simulink model "MR_CIGRE_RESISTIVO"  (R2017b)
settings: Solver=ode23tb  StartTime=0.0  StopTime=t_sim  RelTol=1e-4
values from neighbouring files (symbols this model uses):
  Cdc_Bat1 = 2E-3    (= 0.002)    [Dados_de_Bat_1.m]
  Cf_Bat1 = 5E-6    (= 5e-06)    [Dados_de_Bat_1.m]
  I_max_Bat1 = 1.5*Is_bat1*sqrt(2)    [Dados_de_Bat_1.m]
  Is_bat1 = Sb_Bat1 / (sqrt(3)*Vs2)    [Dados_de_Bat_1.m]
  K_iff_Bat1 = 0    [Dados_de_Bat_1.m]
  Kcij = Rfsj*(2*sig*w_ij*(Tpj + Tfsj)-1)    (= 3.9715)    [Dados_de_Bat_1.m]
  Ki_Bat1 = (R_Bat1+ron_Bat1)/ti_Bat1    (= 201.76)    [Dados_de_Bat_1.m]
  Kp_Bat1 = L_Bat1/ti_Bat1    (= 2.7)    [Dados_de_Bat_1.m]
  Kv_Bat1 = 0.75    [Dados_de_Bat_1.m]
  Kvi_DC = 25*Kvp_DC    (= 7.5)    [Dados_de_Bat_1.m]
  Kvp_DC = 0.3    [Dados_de_Bat_1.m]
  L_10_18 = imag(ug3)*C_10_18    [Dados_de_Linhas.m]
  L_12_13 = imag(ug3)*C_12_13    [Dados_de_Linhas.m]
  L_13_14 = imag(ug3)*C_13_14    [Dados_de_Linhas.m]
  L_14_15 = imag(ug3)*C_14_15    [Dados_de_Linhas.m]
  L_1_2 = imag(ug1)*C_1_2    [Dados_de_Linhas.m]
  L_2_3 = imag(ug1)*C_2_3    [Dados_de_Linhas.m]
  L_3_11 = imag(ug3)*C_3_11    [Dados_de_Linhas.m]
  L_3_4 = imag(ug1)*C_3_4    [Dados_de_Linhas.m]
  L_4_12 = imag(ug3)*C_4_12    [Dados_de_Linhas.m]
  L_4_5 = imag(ug1)*C_4_5    [Dados_de_Linhas.m]
  L_5_6 = imag(ug1)*C_5_6    [Dados_de_Linhas.m]
  L_6_16 = imag(ug3)*C_6_16    [Dados_de_Linhas.m]
  L_6_7 = imag(ug1)*C_6_7    [Dados_de_Linhas.m]
  L_7_8 = imag(ug1)*C_7_8    [Dados_de_Linhas.m]
  L_8_9 = imag(ug1)*C_8_9    [Dados_de_Linhas.m]
  L_9_10 = imag(ug1)*C_9_10    [Dados_de_Linhas.m]
  L_9_17 = imag(ug3)*C_9_17    [Dados_de_Linhas.m]
  L_Bat1 = 1.35E-3    (= 0.00135)    [Dados_de_Bat_1.m]
  L_Bat2 = 1.35E-3    (= 0.00135)    [Dados_de_Bat_2.m]
  L_Virt_Bat1 = 3e-3    (= 0.003)    [Dados_de_Bat_1.m]
  L_Virt_Bat2 = 3.0E-3    (= 0.003)    [Dados_de_Bat_2.m]
  LC_Bat2 = 1e-16    [Dados_de_Bat_2.m]
  Lfsj = 4e-3    (= 0.004)    [Dados_de_Bat_1.m]
  LPF_Ci_Bat1 = 8000    [Dados_de_Bat_1.m]
  LPF_Ci_Bat2 = 5000    [Dados_de_Bat_2.m]
  LPF_Cv_Bat1 = 3000    [Dados_de_Bat_1.m]
  LPF_Q_Bat1 = 3*2*pi()    [Dados_de_Bat_1.m]
  m_Bat1 = 0.05    [Dados_de_Bat_1.m]
  n_Bat1 = 0.05    [Dados_de_Bat_1.m]
  PQ_ref_taxavar_bat1 = 0.5    [Dados_de_Bat_1.m]
  R_10_18 = real(ug3)*C_10_18    [Dados_de_Linhas.m]
  R_12_13 = real(ug3)*C_12_13    [Dados_de_Linhas.m]
  R_13_14 = real(ug3)*C_13_14    [Dados_de_Linhas.m]
  R_14_15 = real(ug3)*C_14_15    [Dados_de_Linhas.m]
  R_1_2 = real(ug1)*C_1_2    [Dados_de_Linhas.m]
  R_2_3 = real(ug1)*C_2_3    [Dados_de_Linhas.m]
  R_3_11 = real(ug3)*C_3_11    [Dados_de_Linhas.m]
  R_3_4 = real(ug1)*C_3_4    [Dados_de_Linhas.m]
  R_4_12 = real(ug3)*C_4_12    [Dados_de_Linhas.m]
  R_4_5 = real(ug1)*C_4_5    [Dados_de_Linhas.m]
  R_5_6 = real(ug1)*C_5_6    [Dados_de_Linhas.m]
  R_6_16 = real(ug3)*C_6_16    [Dados_de_Linhas.m]
  R_6_7 = real(ug1)*C_6_7    [Dados_de_Linhas.m]
  R_7_8 = real(ug1)*C_7_8    [Dados_de_Linhas.m]
  R_8_9 = real(ug1)*C_8_9    [Dados_de_Linhas.m]
  R_9_10 = real(ug1)*C_9_10    [Dados_de_Linhas.m]
  R_9_17 = real(ug3)*C_9_17    [Dados_de_Linhas.m]
  R_Bat1 = 0.1    [Dados_de_Bat_1.m]
  R_Virt_Bat1 = 0    [Dados_de_Bat_1.m]
  R_Virt_Bat2 = 0    [Dados_de_Bat_2.m]
  Rb_bat1 = (N_cell_serie * Rb_cell) / N_string_cell    (= 0.153333333333)    [Dados_de_Bat_1.m]
  RC_Bat2 = 1e-16    [Dados_de_Bat_2.m]
  Rfsj = 0.03    [Dados_de_Bat_1.m]
  ron_Bat1 = 0.88E-3    (= 0.00088)    [Dados_de_Bat_1.m]
  Vdc_Bat1 = 800    [Dados_de_Bat_1.m]
  Voc_bat1 = N_cell_serie * Voc_cell    (= 180)    [Dados_de_Bat_1.m]
  z_Bat1 = z_gk    [Dados_de_Bat_1.m]
undefined symbols (not defined in the file or in its folder): BAT1_CONT, BAT2_CONT, Cdc, Cf, cont_fre, cont_ten, f0, Imax_solar1, Imax_solar2, Ki_interm, Kie, Kiw, Kp_cp, Kp_cr, Kp_interm, Kpe, Kpw, L, LPF_P_Bat1, LPF_P_Interm, LPF_Vdc, P_Solar1, P_Solar2, PQ_ref_time_bat1, Pref_Bat1, Qref_Bat1, Qref_Solar, R, ron, Sb_Bat1, Sb_ger, Sb_sol1, Sb_sol2, t_atraso, t_CS_ini, TDR1, TDR11, TDR15, TDR16, TDR17, TDR18, ti_cp, ti_cr, tilha, TLR11, TLR15, TLR16, TLR17, TLR18, tsinc, Vdc, vref1, Vref_sec, Vs1, Vs2, w0, wref_sec
libraries: powerlib x158, powerlib_meascontrol x59, re_lib x2, simulink x1
(part 4 of 4)

== system MR_CIGRE_RESISTIVO/Banco de Baterias_2/Referencia de  Corrente ==
  Id_feed : Inport
  Iq_feed : Inport  Port=2
  Sw_Mode : Inport  Port=3
  Id_supp : Inport  Port=4
  Iq_supp : Inport  Port=5
  LPF2 : TransferFcn  Denominator=[1/(LPF_Cv_Bat1) 1]
  LPF4 : TransferFcn  Denominator=[1/(LPF_Cv_Bat1) 1]
  Switch : Switch  Criteria=u2 > Threshold
  Switch1 : Switch  Criteria=u2 > Threshold
  Id_ref : Outport
  Iq_ref : Outport  Port=2
  wires:
  Sw_Mode/1 -> Switch/2, Switch1/2
  Switch/1 -> LPF4/1
  Switch1/1 -> LPF2/1
  Id_feed/1 -> Switch/1
  Id_supp/1 -> Switch/3
  Iq_feed/1 -> Switch1/1
  Iq_supp/1 -> Switch1/3
  LPF2/1 -> Iq_ref/1
  LPF4/1 -> Id_ref/1

== system MR_CIGRE_RESISTIVO/Banco de Baterias_2/Referência de Potencia ==
  note: Mudança de referência: no sincronismo (sinc=1)
  note: Ref. Potencia em rampa p.u.
  sinc : Inport
  Pref_bat : Inport  Port=2
  Qref_bat : Inport  Port=3
  Pgd : Inport  Port=4
  Qgd : Inport  Port=5
  Data Store Memory : DataStoreMemory  DataStoreName=Qr  ReadBeforeWriteMsg=warning  WriteAfterWriteMsg=warning  WriteAfterReadMsg=warning  ShowAdditionalParam=off  OutDataTypeStr=double
  Data Store Memory1 : DataStoreMemory  DataStoreName=Pr  ReadBeforeWriteMsg=warning  WriteAfterWriteMsg=warning  WriteAfterReadMsg=warning  VectorParams1D=off  ShowAdditionalParam=off  OutDataTypeStr=double
  Product1 : Product
  Product2 : Product
  Rate Limiter : RateLimiter  RisingSlewLimit=PQ_ref_taxavar_bat1*Sb_Bat1  FallingSlewLimit=-PQ_ref_taxavar_bat1*Sb_Bat1  SampleTimeMode=inherited
  Rate Limiter1 : RateLimiter  RisingSlewLimit=PQ_ref_taxavar_bat1*Sb_Bat1  FallingSlewLimit=-PQ_ref_taxavar_bat1*Sb_Bat1  SampleTimeMode=inherited
  Referência Fonte : MATLAB Function  TreatAsAtomicUnit=on
  Time_init_ref : Step  Time=PQ_ref_time_bat1  SampleTime=0
  Prefbat : Outport
  Qrefbat : Outport  Port=2
  wires:
  Referência Fonte/1(Prefbat) -> Prefbat/1
  Referência Fonte/2(Qrefbat) -> Qrefbat/1
  sinc/1 -> Referência Fonte/5(sinc)
  Pgd/1 -> Referência Fonte/3(p)
  Qgd/1 -> Referência Fonte/4(q)
  Product2/1 -> Rate Limiter1/1
  Time_init_ref/1 -> Product1/2, Product2/1
  Qref_bat/1 -> Product2/2
  Product1/1 -> Rate Limiter/1
  Pref_bat/1 -> Product1/1
  Rate Limiter/1 -> Referência Fonte/1(Pref_bat)
  Rate Limiter1/1 -> Referência Fonte/2(Qref_bat)

== system MR_CIGRE_RESISTIVO/PCC/Ilhamento// Sincronização ==
  sinc : Inport
  Display : Display
  Display1 : Display
  Display3 : Display
  Ilhamento Chave fechada para chave aberta em tilha : Step  Time=tilha  Before=1  After=0  SampleTime=0
  Switch : Switch  Criteria=u2 > Threshold
  sinc=1 : Constant
  "Ch " : Outport
  wires:
  Ilhamento Chave fechada para chave aberta em tilha/1 -> Switch/3, Display3/1
  sinc=1/1 -> Switch/1, Display/1
  Switch/1 -> "Ch "/1, Display1/1
  sinc/1 -> Switch/2

== system MR_CIGRE_RESISTIVO/Sincronização/Microrrede ==
  Vabc : Inport
  Gain4 : Gain  Gain=1/(Vs2*sqrt(2))
  PLL (3ph) : powerlib_meascontrol/PLL/PLL (3ph)  Fmin=45  Par_Init="[0  60]"  ParK=[180, 3200, 1]  TcD=5E-5  MaxRateChangeFreq=12  FilterCutOffFreq=25  Ts=5E-5  AGC=on
  Sequence Analyzer : powerlib_meascontrol/Measurements/Sequence Analyzer  Freq=60  n=1  seq=Positive  InInit=[1, 0]  Ts=0
      settings: SourceProductName=Simscape Power Systems  SourceProductBaseCode=PS
  Ang : Outport
  |V| : Outport  Port=2
  f : Outport  Port=3
  wires:
  Vabc/1 -> Sequence Analyzer/1, PLL (3ph)/1
  PLL (3ph)/1 -> f/1
  Sequence Analyzer/2 -> Ang/1
  Gain4/1 -> |V|/1
  Sequence Analyzer/1 -> Gain4/1

== system MR_CIGRE_RESISTIVO/Sincronização/Rede Principal ==
  Vabc : Inport
  Gain4 : Gain  Gain=1/(Vs2*sqrt(2))
  PLL (3ph) : powerlib_meascontrol/PLL/PLL (3ph)  Fmin=45  Par_Init="[0  60]"  ParK=[180, 3200, 1]  TcD=5E-5  MaxRateChangeFreq=12  FilterCutOffFreq=25  Ts=5E-5  AGC=on
  Sequence Analyzer : powerlib_meascontrol/Measurements/Sequence Analyzer  Freq=60  n=1  seq=Positive  InInit=[1, 0]  Ts=0
      settings: SourceProductName=Simscape Power Systems  SourceProductBaseCode=PS
  f : Outport
  |V| : Outport  Port=2
  Ang : Outport  Port=3
  wires:
  Vabc/1 -> Sequence Analyzer/1, PLL (3ph)/1
  PLL (3ph)/1 -> f/1
  Sequence Analyzer/2 -> Ang/1
  Gain4/1 -> |V|/1
  Sequence Analyzer/1 -> Gain4/1

== system MR_CIGRE_RESISTIVO/Solar_1/Controle Corrente ==
  Idref : Inport
  Iqref : Inport  Port=2
  Vsd : Inport  Port=3
  Vsq : Inport  Port=4
  Id : Inport  Port=5
  Iq : Inport  Port=6
  w : Inport  Port=7
  Vdc/2 : Inport  Port=8
  Controle d : TransferFcn  Numerator=[Kp_interm Ki_interm]  Denominator=[1 0]
  Controle q : TransferFcn  Numerator=[Kp_interm Ki_interm]  Denominator=[1 0]
  Divide : Product  Inputs=*/
  Divide1 : Product  Inputs=/*
  L*w0*Id : Gain  Gain=L_Bat2
  L*w0*Iq : Gain  Gain=L_Bat2
  LPF1 : TransferFcn  Commented=through  Denominator=[1/(LPF_Ci_Bat2) 1]
  LPF2 : TransferFcn  Commented=through  Denominator=[1/(LPF_Ci_Bat2) 1]
  Saturation : Saturate  UpperLimit=1  LowerLimit=-1
  Saturation1 : Saturate  UpperLimit=1  LowerLimit=-1
  Sum1 : Sum  Inputs=-+|
  Sum2 : Sum  Inputs=+|+|-
  Sum3 : Sum  Inputs=|+-
  Sum4 : Sum  Inputs=+|+|+
  d : Product  Inputs=**
  q : Product  Inputs=**
  Md : Outport
  Mq : Outport  Port=2
  wires:
  Vsd/1 -> Sum2/1
  Saturation1/1 -> Md/1
  Saturation/1 -> Mq/1
  Sum2/1 -> Divide/1
  Iq/1 -> d/2, Sum3/2
  Iqref/1 -> Sum3/1
  w/1 -> d/1, q/2
  q/1 -> L*w0*Id/1
  Sum1/1 -> Controle d/1
  L*w0*Iq/1 -> Sum2/3
  Vdc/2/1 -> Divide1/1, Divide/2
  d/1 -> L*w0*Iq/1
  Idref/1 -> Sum1/2
  Sum4/1 -> Divide1/2
  Sum3/1 -> Controle q/1
  Controle d/1 -> Sum2/2
  Controle q/1 -> Sum4/2
  L*w0*Id/1 -> Sum4/1
  Id/1 -> q/1, Sum1/1
  Vsq/1 -> Sum4/3
  Divide1/1 -> LPF1/1
  Divide/1 -> LPF2/1
  LPF2/1 -> Saturation1/1
  LPF1/1 -> Saturation/1

== system MR_CIGRE_RESISTIVO/Solar_1/Controle Potencia  ==
  note: Anti Windup
  note: Anti Windup
  Q_ref : Inport
  Q : Inport  Port=2
  Vdc : Inport  Port=3
  Gain : Gain  Gain=Kp_cp
  Gain1 : Gain  Gain=Kp_cr
  Gain2 : Gain  Gain=Kp_cr
  Gain3 : Gain  Gain=1/Kp_cp
  Gain4 : Gain  Gain=Kp_cp
  Gain5 : Gain  Gain=-1
  Gain6 : Gain  Gain=1/Kp_cp
  Gain7 : Gain  Gain=-1
  Integrador d : TransferFcn  Denominator=[ti_cp 0]
  Integrador d1 : TransferFcn  Denominator=[ti_cr 0]
  Pref1 : Constant  Value=Vdc
  Referencia de  Corrente : Subsystem
  Sum1 : Sum  Inputs=+-|
  Sum10 : Sum  Inputs=+-
  Sum2 : Sum  Inputs=+-|
  Sum3 : Sum  Inputs=||+|+
  Sum4 : Sum  Inputs=+|+||
  Sum5 : Sum  Inputs=+|-
  Sum6 : Sum  Inputs=-+
  Sum8 : Sum  Inputs=+|-
  Id_ref : Outport
  Iq_ref : Outport  Port=2
  wires:
  Vdc/1 -> Sum1/2
  Pref1/1 -> Sum1/1
  Integrador d1/1 -> Sum3/2
  Sum2/1 -> Gain5/1
  Q_ref/1 -> Sum2/1
  Q/1 -> Sum2/2
  Gain3/1 -> Sum6/1
  Referencia de  Corrente/1(Id_lim) -> Id_ref/1, Sum5/2
  Sum4/1 -> Sum5/1, Referencia de  Corrente/1(Id_ref)
  Gain6/1 -> Sum10/2
  Sum8/1 -> Gain6/1
  Sum5/1 -> Gain3/1
  Referencia de  Corrente/2(Iq_lim) -> Iq_ref/1, Sum8/2
  Sum3/1 -> Referencia de  Corrente/2(Iq_ref), Sum8/1
  Gain1/1 -> Integrador d1/1
  Sum10/1 -> Gain1/1
  Gain2/1 -> Sum3/1
  Gain/1 -> Integrador d/1
  Sum6/1 -> Gain/1
  Sum1/1 -> Gain7/1
  Gain4/1 -> Sum4/2
  Gain5/1 -> Gain2/1, Sum10/1
  Gain7/1 -> Gain4/1, Sum6/2
  Integrador d/1 -> Sum4/1

== system MR_CIGRE_RESISTIVO/Solar_1/Elo CC ==
  CM1 : powerlib/Measurements/Current Measurement  PhasorSimulation=off  OutputType=Complex  PSBequivalent=0
  P : Product  Inputs=**
  Parallel RLC Branch : powerlib/Elements/Parallel RLC Branch  LConnTagsString=a  RConnTagsString=__new0  BranchType=C  Resistance=10000000  Inductance=0  SetiL0=off  InitialCurrent=0  Capacitance=Cdc  Setx0=on  InitialVoltage=710  Measurements=None
  Unit Delay1 : UnitDelay  Commented=through  InitialCondition=700  SampleTime=1E-6
  VM1 : powerlib/Measurements/Voltage Measurement  PhasorSimulation=off  OutputType=Complex  PSBequivalent=0
  + in : PMIOPort  Port=1  Side=Left
  - in : PMIOPort  Port=2  Side=Left
  + out : PMIOPort  Port=3  Side=Right
  - out : PMIOPort  Port=4  Side=Right
  Vdc : Outport
  Pout : Outport  Port=2
  wires:
  VM1/1 -> P/2, Unit Delay1/1
  P/1 -> Pout/1
  CM1/1 -> P/1
  Unit Delay1/1 -> Vdc/1
  connections:
  VM1/LConn2 -- - out/RConn1 -- Parallel RLC Branch/RConn1 -- - in/RConn1
  VM1/LConn1 -- CM1/LConn1 -- + in/RConn1 -- Parallel RLC Branch/LConn1
  + out/RConn1 -- CM1/RConn1

== system MR_CIGRE_RESISTIVO/Solar_1/Fonte Fotovoltaica ==
  CM1 : powerlib/Measurements/Current Measurement  PhasorSimulation=off  OutputType=Complex  PSBequivalent=0
  P : Product  Inputs=**
  PV Array : re_lib/Solar/PV Array  Npar=P_Solar1/3000  Nser=10  PlotType=array @ 1000 W/m2 & specified temperatures  S_vec="[ 1000  500  100 ]"  Temp_C_vec="[ 45 25  ]"  ModuleName=Canadian Solar CS6X-300P  PlotWhenSelected=off  Pm=299.63  Ncell=72  Voc=44.6  Isc=8.87  Vm=36.1  Im=8.3  beta_Voc_pc=-0.395  alpha_Isc_pc=0.052999  beta_Voc=-0.17617  alpha_Isc=0.004701  IL=8.9088  I0=9.446e-10  nI=1.0506  Rsh=262.4171  Rs=0.34354  BAL=off  Tc=1e-6  Tfilter=5e-5
  Pref3 : Constant  Value=1000
  Pref4 : Constant  Value=25
  Pref5 : Constant  Value=0.5157
  Two-Quadrant DC/DC Converter : powerlib/Power Electronics/Two-Quadrant DC//DC Converter  ModelType=Average model (D-controlled)  Ron=1e-3  Rs=1e6  Cs=inf  Vforward=[0,0]  Ron_Diode=1e-3  Rs_Diode=1e6  Cs_Diode=inf  Vf_Diode=1e-3  Rs_CurrentSource=inf
      settings: SourceProductName=Simscape Power Systems  SourceProductBaseCode=PS
  VM1 : powerlib/Measurements/Voltage Measurement  PhasorSimulation=off  OutputType=Complex  PSBequivalent=0
  VM3 : powerlib/Measurements/Voltage Measurement  PhasorSimulation=off  OutputType=Complex  PSBequivalent=0
  w3 : Scope
  + out : PMIOPort  Port=1  Side=Left
  - out : PMIOPort  Port=2  Side=Left
  V_fv : Outport
  P_fv : Outport  Port=2
  wires:
  Pref3/1 -> PV Array/1
  Pref5/1 -> Two-Quadrant DC/DC Converter/1
  VM3/1 -> w3/1
  Pref4/1 -> PV Array/2
  VM1/1 -> V_fv/1, P/2
  CM1/1 -> P/1
  P/1 -> P_fv/1
  connections:
  PV Array/RConn2 -- VM3/LConn2 -- VM1/LConn2 -- - out/RConn1 -- Two-Quadrant DC/DC Converter/RConn2
  VM3/LConn1 -- PV Array/RConn1 -- Two-Quadrant DC/DC Converter/LConn1
  CM1/LConn1 -- Two-Quadrant DC/DC Converter/RConn1
  + out/RConn1 -- VM1/LConn1 -- CM1/RConn1

== system MR_CIGRE_RESISTIVO/Solar_1/Fonte de Tensão 3f2 ==
  Vabc : Inport
  R+ron+L VSC1 : powerlib/Elements/Three-Phase Series RLC Branch  LConnTagsString=A|B|C  RConnTagsString=A|B|C  BranchType=RL  Resistance=R+ron  Inductance=L  Capacitance=1e-6  Measurements=None
  Sequence Analyzer5 : powerlib_meascontrol/Measurements/Sequence Analyzer  Commented=on  Freq=60  n=1  seq=Positive  InInit=[1, 0]  Ts=0
      settings: SourceProductName=Simscape Power Systems  SourceProductBaseCode=PS
  Three-Phase Series RLC Branch2 : powerlib/Elements/Three-Phase Series RLC Branch  LConnTagsString=A|B|C  RConnTagsString=A|B|C  BranchType=C  Resistance=1  Inductance=1e-3  Capacitance=Cf  Measurements=None
  V&I - VSC2 2 : powerlib/Measurements/Three-Phase V-I Measurement  VoltageMeasurement=phase-to-ground  SetLabelV=off  LabelV=Vabc  Vpu=off  VpuLL=off  CurrentMeasurement=yes  SetLabelI=off  LabelI=Iabc  Ipu=off  Pbase=100e6  Vbase=500e3  OutputType=Complex  PhasorSimulation=off  PSBequivalent=0
  VSC (Average Model) : powerlib/Power Electronics/Universal Bridge  Arms=3  SnubberResistance=1e5  SnubberCapacitance=inf  Device=Average-model based VSC  Ron=1e-3  Lon=0  ForwardVoltages="[  0  0  ]"  ForwardVoltage=0  GTOparameters=[ 10e-6 , 20e-6 ]  IGBTparameters=[ 1e-6 , 2e-6 ]  Measurements=None  Measurements_2=None  converterType=Rectifier
  m3 : Scope  Commented=on  NumInputPorts=2
  Va : PMIOPort  Port=1  Side=Right
  Vb : PMIOPort  Port=2  Side=Right
  Vc : PMIOPort  Port=3  Side=Right
  GND : PMIOPort  Port=4  Side=Right
  + : PMIOPort  Port=5  Side=Left
  - : PMIOPort  Port=6  Side=Left
  Vabc_M : Outport
  Iabc_M : Outport  Port=2
  wires:
  V&I - VSC2 2/1 -> Vabc_M/1
  V&I - VSC2 2/2 -> Iabc_M/1
  Vabc/1 -> Sequence Analyzer5/1, VSC (Average Model)/1
  Sequence Analyzer5/1 -> m3/1
  Sequence Analyzer5/2 -> m3/2
  connections:
  Three-Phase Series RLC Branch2/RConn2 -- Three-Phase Series RLC Branch2/RConn1 -- GND/RConn1 -- Three-Phase Series RLC Branch2/RConn3
  R+ron+L VSC1/LConn1 -- V&I - VSC2 2/RConn1
  R+ron+L VSC1/LConn2 -- V&I - VSC2 2/RConn2
  R+ron+L VSC1/LConn3 -- V&I - VSC2 2/RConn3
  Three-Phase Series RLC Branch2/LConn1 -- Va/RConn1 -- R+ron+L VSC1/RConn1
  Three-Phase Series RLC Branch2/LConn2 -- Vb/RConn1 -- R+ron+L VSC1/RConn2
  Three-Phase Series RLC Branch2/LConn3 -- Vc/RConn1 -- R+ron+L VSC1/RConn3
  VSC (Average Model)/LConn1 -- V&I - VSC2 2/LConn1
  VSC (Average Model)/LConn2 -- V&I - VSC2 2/LConn2
  VSC (Average Model)/LConn3 -- V&I - VSC2 2/LConn3
  +/RConn1 -- VSC (Average Model)/RConn1
  -/RConn1 -- VSC (Average Model)/RConn2

== system MR_CIGRE_RESISTIVO/Solar_1/Medidor de pot ==
  Vd : Inport
  Vq : Inport  Port=2
  Id : Inport  Port=3
  Iq : Inport  Port=4
  Gain : Gain  Gain=1.5
  Gain1 : Gain  Gain=1.5
  Sum1 : Sum  Inputs=+|+
  Sum2 : Sum  Inputs=-|+
  a : Product  Inputs=**
  a1 : Product  Inputs=**
  b1 : Product  Inputs=**
  b2 : Product  Inputs=**
  P : Outport
  Q : Outport  Port=2
  wires:
  a1/1 -> Sum1/2
  Vq/1 -> b2/2, a1/1
  a/1 -> Sum1/1
  b1/1 -> Sum2/1
  Sum1/1 -> Gain/1
  b2/1 -> Sum2/2
  Iq/1 -> b1/2, a1/2
  Vd/1 -> b1/1, a/1
  Id/1 -> b2/1, a/2
  Sum2/1 -> Gain1/1
  Gain/1 -> P/1
  Gain1/1 -> Q/1

== system MR_CIGRE_RESISTIVO/Solar_1/PLL e Medidor1 ==
  note: Medida de w e wt do Sistema
  note: Medida Vd, Vq, Iq e Id
  Iabc_M : Inport
  Iabc_S : Inport  Port=2
  Vabc_S : Inport  Port=3
  wt : Inport  Port=4
  2*pi()*f : Gain  Gain=2*pi()
  Iabc-Idq : powerlib_meascontrol/Transformations/abc to dq0  Alignment=90 degrees behind phase A axis
  Iabc-Idq1 : powerlib_meascontrol/Transformations/abc to dq0  Alignment=90 degrees behind phase A axis
  Iabc-Idq2 : powerlib_meascontrol/Transformations/abc to dq0  Alignment=90 degrees behind phase A axis
  PLL (3ph) : powerlib_meascontrol/PLL/PLL (3ph)  Fmin=1  Par_Init="[0  f0]"  ParK=[180, 3200, 1]  TcD=5E-5  MaxRateChangeFreq=120  FilterCutOffFreq=25  Ts=5E-5  AGC=on
  Sys_wt : Outport
  Sys_w : Outport  Port=2
  Vdq0_S : Outport  Port=3
  Idq_M : Outport  Port=4
  Idq0_S : Outport  Port=5
  wires:
  PLL (3ph)/1 -> 2*pi()*f/1
  Iabc_S/1 -> Iabc-Idq/1
  Vabc_S/1 -> Iabc-Idq1/1, PLL (3ph)/1
  Iabc_M/1 -> Iabc-Idq2/1
  Iabc-Idq/1 -> Idq0_S/1
  Iabc-Idq2/1 -> Idq_M/1
  Iabc-Idq1/1 -> Vdq0_S/1
  2*pi()*f/1 -> Sys_w/1
  wt/1 -> [wt]
  PLL (3ph)/2 -> Sys_wt/1
  [wt] -> Iabc-Idq1/2
  [wt] -> Iabc-Idq2/2
  [wt] -> Iabc-Idq/2

== system MR_CIGRE_RESISTIVO/Solar_2/Controle Corrente ==
  Idref : Inport
  Iqref : Inport  Port=2
  Vsd : Inport  Port=3
  Vsq : Inport  Port=4
  Id : Inport  Port=5
  Iq : Inport  Port=6
  w : Inport  Port=7
  Vdc/2 : Inport  Port=8
  Controle d : TransferFcn  Numerator=[Kp_interm Ki_interm]  Denominator=[1 0]
  Controle q : TransferFcn  Numerator=[Kp_interm Ki_interm]  Denominator=[1 0]
  Divide : Product  Inputs=*/
  Divide1 : Product  Inputs=/*
  L*w0*Id : Gain  Gain=L_Bat2
  L*w0*Iq : Gain  Gain=L_Bat2
  LPF1 : TransferFcn  Commented=through  Denominator=[1/(LPF_Ci_Bat2) 1]
  LPF2 : TransferFcn  Commented=through  Denominator=[1/(LPF_Ci_Bat2) 1]
  Saturation : Saturate  UpperLimit=1  LowerLimit=-1
  Saturation1 : Saturate  UpperLimit=1  LowerLimit=-1
  Sum1 : Sum  Inputs=-+|
  Sum2 : Sum  Inputs=+|+|-
  Sum3 : Sum  Inputs=|+-
  Sum4 : Sum  Inputs=+|+|+
  d : Product  Inputs=**
  q : Product  Inputs=**
  Md : Outport
  Mq : Outport  Port=2
  wires:
  Vsd/1 -> Sum2/1
  Saturation1/1 -> Md/1
  Saturation/1 -> Mq/1
  Sum2/1 -> Divide/1
  Iq/1 -> d/2, Sum3/2
  Iqref/1 -> Sum3/1
  w/1 -> d/1, q/2
  q/1 -> L*w0*Id/1
  Sum1/1 -> Controle d/1
  L*w0*Iq/1 -> Sum2/3
  Vdc/2/1 -> Divide1/1, Divide/2
  d/1 -> L*w0*Iq/1
  Idref/1 -> Sum1/2
  Sum4/1 -> Divide1/2
  Sum3/1 -> Controle q/1
  Controle d/1 -> Sum2/2
  Controle q/1 -> Sum4/2
  L*w0*Id/1 -> Sum4/1
  Id/1 -> q/1, Sum1/1
  Vsq/1 -> Sum4/3
  Divide1/1 -> LPF1/1
  Divide/1 -> LPF2/1
  LPF2/1 -> Saturation1/1
  LPF1/1 -> Saturation/1

== system MR_CIGRE_RESISTIVO/Solar_2/Controle Potencia  ==
  note: Anti Windup
  note: Anti Windup
  Q_ref : Inport
  Q : Inport  Port=2
  Vdc : Inport  Port=3
  Gain : Gain  Gain=Kp_cp
  Gain1 : Gain  Gain=Kp_cr
  Gain2 : Gain  Gain=Kp_cr
  Gain3 : Gain  Gain=1/Kp_cp
  Gain4 : Gain  Gain=Kp_cp
  Gain5 : Gain  Gain=-1
  Gain6 : Gain  Gain=1/Kp_cp
  Gain7 : Gain  Gain=-1
  Integrador d : TransferFcn  Denominator=[ti_cp 0]
  Integrador d1 : TransferFcn  Denominator=[ti_cr 0]
  Pref1 : Constant  Value=Vdc
  Referencia de  Corrente : Subsystem
  Sum1 : Sum  Inputs=+-|
  Sum10 : Sum  Inputs=+-
  Sum2 : Sum  Inputs=+-|
  Sum3 : Sum  Inputs=||+|+
  Sum4 : Sum  Inputs=+|+||
  Sum5 : Sum  Inputs=+|-
  Sum6 : Sum  Inputs=-+
  Sum8 : Sum  Inputs=+|-
  Id_ref : Outport
  Iq_ref : Outport  Port=2
  wires:
  Vdc/1 -> Sum1/2
  Pref1/1 -> Sum1/1
  Integrador d1/1 -> Sum3/2
  Sum2/1 -> Gain5/1
  Q_ref/1 -> Sum2/1
  Q/1 -> Sum2/2
  Gain3/1 -> Sum6/1
  Referencia de  Corrente/1(Id_lim) -> Id_ref/1, Sum5/2
  Sum4/1 -> Sum5/1, Referencia de  Corrente/1(Id_ref)
  Gain6/1 -> Sum10/2
  Sum8/1 -> Gain6/1
  Sum5/1 -> Gain3/1
  Referencia de  Corrente/2(Iq_lim) -> Iq_ref/1, Sum8/2
  Sum3/1 -> Referencia de  Corrente/2(Iq_ref), Sum8/1
  Gain1/1 -> Integrador d1/1
  Sum10/1 -> Gain1/1
  Gain2/1 -> Sum3/1
  Gain/1 -> Integrador d/1
  Sum6/1 -> Gain/1
  Sum1/1 -> Gain7/1
  Gain4/1 -> Sum4/2
  Gain5/1 -> Gain2/1, Sum10/1
  Gain7/1 -> Gain4/1, Sum6/2
  Integrador d/1 -> Sum4/1

== system MR_CIGRE_RESISTIVO/Solar_2/Elo CC ==
  CM1 : powerlib/Measurements/Current Measurement  PhasorSimulation=off  OutputType=Complex  PSBequivalent=0
  P : Product  Inputs=**
  Parallel RLC Branch : powerlib/Elements/Parallel RLC Branch  LConnTagsString=a  RConnTagsString=__new0  BranchType=C  Resistance=10000000  Inductance=0  SetiL0=off  InitialCurrent=0  Capacitance=Cdc  Setx0=on  InitialVoltage=710  Measurements=None
  Unit Delay1 : UnitDelay  Commented=through  InitialCondition=700  SampleTime=1E-6
  VM1 : powerlib/Measurements/Voltage Measurement  PhasorSimulation=off  OutputType=Complex  PSBequivalent=0
  + in : PMIOPort  Port=1  Side=Left
  - in : PMIOPort  Port=2  Side=Left
  + out : PMIOPort  Port=3  Side=Right
  - out : PMIOPort  Port=4  Side=Right
  Vdc : Outport
  Pout : Outport  Port=2
  wires:
  VM1/1 -> P/2, Unit Delay1/1
  P/1 -> Pout/1
  CM1/1 -> P/1
  Unit Delay1/1 -> Vdc/1
  connections:
  VM1/LConn2 -- - out/RConn1 -- Parallel RLC Branch/RConn1 -- - in/RConn1
  VM1/LConn1 -- CM1/LConn1 -- + in/RConn1 -- Parallel RLC Branch/LConn1
  + out/RConn1 -- CM1/RConn1

== system MR_CIGRE_RESISTIVO/Solar_2/Fonte Fotovoltaica ==
  CM1 : powerlib/Measurements/Current Measurement  PhasorSimulation=off  OutputType=Complex  PSBequivalent=0
  P : Product  Inputs=**
  PV Array : re_lib/Solar/PV Array  Npar=P_Solar2/3000  Nser=10  PlotType=array @ 1000 W/m2 & specified temperatures  S_vec="[ 1000  500  100 ]"  Temp_C_vec="[ 45 25  ]"  ModuleName=Canadian Solar CS6X-300P  PlotWhenSelected=off  Pm=299.63  Ncell=72  Voc=44.6  Isc=8.87  Vm=36.1  Im=8.3  beta_Voc_pc=-0.395  alpha_Isc_pc=0.052999  beta_Voc=-0.17617  alpha_Isc=0.004701  IL=8.9088  I0=9.446e-10  nI=1.0506  Rsh=262.4171  Rs=0.34354  BAL=off  Tc=1e-6  Tfilter=5e-5
  Pref3 : Constant  Value=1000
  Pref4 : Constant  Value=25
  Pref5 : Constant  Value=0.5157
  Two-Quadrant DC/DC Converter : powerlib/Power Electronics/Two-Quadrant DC//DC Converter  ModelType=Average model (D-controlled)  Ron=1e-3  Rs=1e6  Cs=inf  Vforward=[0,0]  Ron_Diode=1e-3  Rs_Diode=1e6  Cs_Diode=inf  Vf_Diode=1e-3  Rs_CurrentSource=inf
      settings: SourceProductName=Simscape Power Systems  SourceProductBaseCode=PS
  VM1 : powerlib/Measurements/Voltage Measurement  PhasorSimulation=off  OutputType=Complex  PSBequivalent=0
  VM3 : powerlib/Measurements/Voltage Measurement  PhasorSimulation=off  OutputType=Complex  PSBequivalent=0
  w3 : Scope
  + out : PMIOPort  Port=1  Side=Left
  - out : PMIOPort  Port=2  Side=Left
  V_fv : Outport
  P_fv : Outport  Port=2
  wires:
  Pref3/1 -> PV Array/1
  Pref5/1 -> Two-Quadrant DC/DC Converter/1
  VM3/1 -> w3/1
  Pref4/1 -> PV Array/2
  VM1/1 -> V_fv/1, P/2
  CM1/1 -> P/1
  P/1 -> P_fv/1
  connections:
  PV Array/RConn2 -- VM3/LConn2 -- VM1/LConn2 -- - out/RConn1 -- Two-Quadrant DC/DC Converter/RConn2
  VM3/LConn1 -- PV Array/RConn1 -- Two-Quadrant DC/DC Converter/LConn1
  CM1/LConn1 -- Two-Quadrant DC/DC Converter/RConn1
  + out/RConn1 -- VM1/LConn1 -- CM1/RConn1

== system MR_CIGRE_RESISTIVO/Solar_2/Fonte de Tensão 3f2 ==
  Vabc : Inport
  R+ron+L VSC1 : powerlib/Elements/Three-Phase Series RLC Branch  LConnTagsString=A|B|C  RConnTagsString=A|B|C  BranchType=RL  Resistance=R+ron  Inductance=L  Capacitance=1e-6  Measurements=None
  Sequence Analyzer5 : powerlib_meascontrol/Measurements/Sequence Analyzer  Commented=on  Freq=60  n=1  seq=Positive  InInit=[1, 0]  Ts=0
      settings: SourceProductName=Simscape Power Systems  SourceProductBaseCode=PS
  Three-Phase Series RLC Branch2 : powerlib/Elements/Three-Phase Series RLC Branch  LConnTagsString=A|B|C  RConnTagsString=A|B|C  BranchType=C  Resistance=1  Inductance=1e-3  Capacitance=Cf  Measurements=None
  V&I - VSC2 2 : powerlib/Measurements/Three-Phase V-I Measurement  VoltageMeasurement=phase-to-ground  SetLabelV=off  LabelV=Vabc  Vpu=off  VpuLL=off  CurrentMeasurement=yes  SetLabelI=off  LabelI=Iabc  Ipu=off  Pbase=100e6  Vbase=500e3  OutputType=Complex  PhasorSimulation=off  PSBequivalent=0
  VSC (Average Model) : powerlib/Power Electronics/Universal Bridge  Arms=3  SnubberResistance=1e5  SnubberCapacitance=inf  Device=Average-model based VSC  Ron=1e-3  Lon=0  ForwardVoltages="[  0  0  ]"  ForwardVoltage=0  GTOparameters=[ 10e-6 , 20e-6 ]  IGBTparameters=[ 1e-6 , 2e-6 ]  Measurements=None  Measurements_2=None  converterType=Rectifier
  m3 : Scope  Commented=on  NumInputPorts=2
  Va : PMIOPort  Port=1  Side=Right
  Vb : PMIOPort  Port=2  Side=Right
  Vc : PMIOPort  Port=3  Side=Right
  GND : PMIOPort  Port=4  Side=Right
  + : PMIOPort  Port=5  Side=Left
  - : PMIOPort  Port=6  Side=Left
  Vabc_M : Outport
  Iabc_M : Outport  Port=2
  wires:
  V&I - VSC2 2/1 -> Vabc_M/1
  V&I - VSC2 2/2 -> Iabc_M/1
  Vabc/1 -> Sequence Analyzer5/1, VSC (Average Model)/1
  Sequence Analyzer5/1 -> m3/1
  Sequence Analyzer5/2 -> m3/2
  connections:
  Three-Phase Series RLC Branch2/RConn2 -- Three-Phase Series RLC Branch2/RConn1 -- GND/RConn1 -- Three-Phase Series RLC Branch2/RConn3
  R+ron+L VSC1/LConn1 -- V&I - VSC2 2/RConn1
  R+ron+L VSC1/LConn2 -- V&I - VSC2 2/RConn2
  R+ron+L VSC1/LConn3 -- V&I - VSC2 2/RConn3
  Three-Phase Series RLC Branch2/LConn1 -- Va/RConn1 -- R+ron+L VSC1/RConn1
  Three-Phase Series RLC Branch2/LConn2 -- Vb/RConn1 -- R+ron+L VSC1/RConn2
  Three-Phase Series RLC Branch2/LConn3 -- Vc/RConn1 -- R+ron+L VSC1/RConn3
  VSC (Average Model)/LConn1 -- V&I - VSC2 2/LConn1
  VSC (Average Model)/LConn2 -- V&I - VSC2 2/LConn2
  VSC (Average Model)/LConn3 -- V&I - VSC2 2/LConn3
  +/RConn1 -- VSC (Average Model)/RConn1
  -/RConn1 -- VSC (Average Model)/RConn2

== system MR_CIGRE_RESISTIVO/Solar_2/Medidor de pot ==
  Vd : Inport
  Vq : Inport  Port=2
  Id : Inport  Port=3
  Iq : Inport  Port=4
  Gain : Gain  Gain=1.5
  Gain1 : Gain  Gain=1.5
  Sum1 : Sum  Inputs=+|+
  Sum2 : Sum  Inputs=-|+
  a : Product  Inputs=**
  a1 : Product  Inputs=**
  b1 : Product  Inputs=**
  b2 : Product  Inputs=**
  P : Outport
  Q : Outport  Port=2
  wires:
  a1/1 -> Sum1/2
  Vq/1 -> b2/2, a1/1
  a/1 -> Sum1/1
  b1/1 -> Sum2/1
  Sum1/1 -> Gain/1
  b2/1 -> Sum2/2
  Iq/1 -> b1/2, a1/2
  Vd/1 -> b1/1, a/1
  Id/1 -> b2/1, a/2
  Sum2/1 -> Gain1/1
  Gain/1 -> P/1
  Gain1/1 -> Q/1

== system MR_CIGRE_RESISTIVO/Solar_2/PLL e Medidor1 ==
  note: Medida de w e wt do Sistema
  note: Medida Vd, Vq, Iq e Id
  Iabc_M : Inport
  Iabc_S : Inport  Port=2
  Vabc_S : Inport  Port=3
  wt : Inport  Port=4
  2*pi()*f : Gain  Gain=2*pi()
  Iabc-Idq : powerlib_meascontrol/Transformations/abc to dq0  Alignment=90 degrees behind phase A axis
  Iabc-Idq1 : powerlib_meascontrol/Transformations/abc to dq0  Alignment=90 degrees behind phase A axis
  Iabc-Idq2 : powerlib_meascontrol/Transformations/abc to dq0  Alignment=90 degrees behind phase A axis
  PLL (3ph) : powerlib_meascontrol/PLL/PLL (3ph)  Fmin=1  Par_Init="[0  f0]"  ParK=[180, 3200, 1]  TcD=5E-5  MaxRateChangeFreq=120  FilterCutOffFreq=25  Ts=5E-5  AGC=on
  Sys_wt : Outport
  Sys_w : Outport  Port=2
  Vdq0_S : Outport  Port=3
  Idq_M : Outport  Port=4
  Idq0_S : Outport  Port=5
  wires:
  PLL (3ph)/1 -> 2*pi()*f/1
  Iabc_S/1 -> Iabc-Idq/1
  Vabc_S/1 -> Iabc-Idq1/1, PLL (3ph)/1
  Iabc_M/1 -> Iabc-Idq2/1
  Iabc-Idq/1 -> Idq0_S/1
  Iabc-Idq2/1 -> Idq_M/1
  Iabc-Idq1/1 -> Vdq0_S/1
  2*pi()*f/1 -> Sys_w/1
  wt/1 -> [wt]
  PLL (3ph)/2 -> Sys_wt/1
  [wt] -> Iabc-Idq1/2
  [wt] -> Iabc-Idq2/2
  [wt] -> Iabc-Idq/2

== system MR_CIGRE_RESISTIVO/Banco de Baterias_1/Controle Corrente/Limite Corrente ==
  Id : Inport
  Iq : Inport  Port=2
  Complex to Magnitude-Angle : ComplexToMagnitudeAngle
  Complex to Real-Imag : ComplexToRealImag
  Magnitude-Angle to Complex : MagnitudeAngleToComplex
  Real-Imag to Complex : RealImagToComplex
  Saturation : Saturate  UpperLimit=1  LowerLimit=-1
  Id_lim : Outport
  Iq_lim : Outport  Port=2
  wires:
  Complex to Magnitude-Angle/1 -> Saturation/1
  Magnitude-Angle to Complex/1 -> Complex to Real-Imag/1
  Id/1 -> Real-Imag to Complex/1
  Saturation/1 -> Magnitude-Angle to Complex/1
  Complex to Real-Imag/1 -> Id_lim/1
  Complex to Magnitude-Angle/2 -> Magnitude-Angle to Complex/2
  Real-Imag to Complex/1 -> Complex to Magnitude-Angle/1
  Complex to Real-Imag/2 -> Iq_lim/1
  Iq/1 -> Real-Imag to Complex/2

== system MR_CIGRE_RESISTIVO/Banco de Baterias_1/Controle de Tensao/Limite Corrente ==
  Id : Inport
  Iq : Inport  Port=2
  Complex to Magnitude-Angle : ComplexToMagnitudeAngle
  Complex to Real-Imag : ComplexToRealImag
  Magnitude-Angle to Complex : MagnitudeAngleToComplex
  Real-Imag to Complex : RealImagToComplex
  Saturation : Saturate  UpperLimit=I_max_Bat1  LowerLimit=-I_max_Bat1
  Id_lim : Outport
  Iq_lim : Outport  Port=2
  wires:
  Complex to Magnitude-Angle/1 -> Saturation/1
  Magnitude-Angle to Complex/1 -> Complex to Real-Imag/1
  Id/1 -> Real-Imag to Complex/1
  Saturation/1 -> Magnitude-Angle to Complex/1
  Complex to Real-Imag/1 -> Id_lim/1
  Complex to Magnitude-Angle/2 -> Magnitude-Angle to Complex/2
  Real-Imag to Complex/1 -> Complex to Magnitude-Angle/1
  Complex to Real-Imag/2 -> Iq_lim/1
  Iq/1 -> Real-Imag to Complex/2

== system MR_CIGRE_RESISTIVO/Banco de Baterias_1/Controle de potência modo conectado/Subsystem ==
  In1 : Inport
  Demux2 : Demux  Outputs=3
  LPF1 : TransferFcn  Numerator=[0 1]  Denominator=[1/(60*2*pi()) 1]
  LPF2 : TransferFcn  Numerator=[0 1]  Denominator=[1/(60*2*pi()) 1]
  LPF3 : TransferFcn  Numerator=[0 1]  Denominator=[1/(60*2*pi()) 1]
  Mux : Mux  Inputs=3
  Out1 : Outport
  wires:
  Demux2/1 -> LPF3/1
  LPF1/1 -> Mux/2
  LPF3/1 -> Mux/1
  LPF2/1 -> Mux/3
  Demux2/3 -> LPF2/1
  Demux2/2 -> LPF1/1
  In1/1 -> Demux2/1
  Mux/1 -> Out1/1

== system MR_CIGRE_RESISTIVO/Banco de Baterias_2/Controle Corrente/Limite Corrente ==
  Id : Inport
  Iq : Inport  Port=2
  Complex to Magnitude-Angle : ComplexToMagnitudeAngle
  Complex to Real-Imag : ComplexToRealImag
  Magnitude-Angle to Complex : MagnitudeAngleToComplex
  Real-Imag to Complex : RealImagToComplex
  Saturation : Saturate  UpperLimit=1  LowerLimit=-1
  Id_lim : Outport
  Iq_lim : Outport  Port=2
  wires:
  Complex to Magnitude-Angle/1 -> Saturation/1
  Magnitude-Angle to Complex/1 -> Complex to Real-Imag/1
  Id/1 -> Real-Imag to Complex/1
  Saturation/1 -> Magnitude-Angle to Complex/1
  Complex to Real-Imag/1 -> Id_lim/1
  Complex to Magnitude-Angle/2 -> Magnitude-Angle to Complex/2
  Real-Imag to Complex/1 -> Complex to Magnitude-Angle/1
  Complex to Real-Imag/2 -> Iq_lim/1
  Iq/1 -> Real-Imag to Complex/2

== system MR_CIGRE_RESISTIVO/Banco de Baterias_2/Controle de Tensao/Limite Corrente ==
  Id : Inport
  Iq : Inport  Port=2
  Complex to Magnitude-Angle : ComplexToMagnitudeAngle
  Complex to Real-Imag : ComplexToRealImag
  Magnitude-Angle to Complex : MagnitudeAngleToComplex
  Real-Imag to Complex : RealImagToComplex
  Saturation : Saturate  UpperLimit=I_max_Bat1  LowerLimit=-I_max_Bat1
  Id_lim : Outport
  Iq_lim : Outport  Port=2
  wires:
  Complex to Magnitude-Angle/1 -> Saturation/1
  Magnitude-Angle to Complex/1 -> Complex to Real-Imag/1
  Id/1 -> Real-Imag to Complex/1
  Saturation/1 -> Magnitude-Angle to Complex/1
  Complex to Real-Imag/1 -> Id_lim/1
  Complex to Magnitude-Angle/2 -> Magnitude-Angle to Complex/2
  Real-Imag to Complex/1 -> Complex to Magnitude-Angle/1
  Complex to Real-Imag/2 -> Iq_lim/1
  Iq/1 -> Real-Imag to Complex/2

== system MR_CIGRE_RESISTIVO/Banco de Baterias_2/Controle de potência modo conectado/Subsystem ==
  In1 : Inport
  Demux2 : Demux  Outputs=3
  LPF1 : TransferFcn  Numerator=[0 1]  Denominator=[1/(60*2*pi()) 1]
  LPF2 : TransferFcn  Numerator=[0 1]  Denominator=[1/(60*2*pi()) 1]
  LPF3 : TransferFcn  Numerator=[0 1]  Denominator=[1/(60*2*pi()) 1]
  Mux : Mux  Inputs=3
  Out1 : Outport
  wires:
  Demux2/1 -> LPF3/1
  LPF1/1 -> Mux/2
  LPF3/1 -> Mux/1
  LPF2/1 -> Mux/3
  Demux2/3 -> LPF2/1
  Demux2/2 -> LPF1/1
  In1/1 -> Demux2/1
  Mux/1 -> Out1/1

== system MR_CIGRE_RESISTIVO/Solar_1/Controle Potencia /Referencia de  Corrente ==
  Id_ref : Inport
  Iq_ref : Inport  Port=2
  Complex to Magnitude-Angle : ComplexToMagnitudeAngle
  Complex to Real-Imag : ComplexToRealImag
  Magnitude-Angle to Complex : MagnitudeAngleToComplex
  Real-Imag to Complex : RealImagToComplex
  Saturation : Saturate  UpperLimit=Imax_solar1  LowerLimit=-Imax_solar1
  w3 : Scope  NumInputPorts=2
  Id_lim : Outport
  Iq_lim : Outport  Port=2
  wires:
  Complex to Magnitude-Angle/2 -> Magnitude-Angle to Complex/2
  Magnitude-Angle to Complex/1 -> Complex to Real-Imag/1
  Iq_ref/1 -> Real-Imag to Complex/2
  Id_ref/1 -> Real-Imag to Complex/1
  Complex to Magnitude-Angle/1 -> w3/1, Saturation/1
  Real-Imag to Complex/1 -> Complex to Magnitude-Angle/1
  Complex to Real-Imag/1 -> Id_lim/1
  Complex to Real-Imag/2 -> Iq_lim/1
  Saturation/1 -> w3/2, Magnitude-Angle to Complex/1

== system MR_CIGRE_RESISTIVO/Solar_2/Controle Potencia /Referencia de  Corrente ==
  Id_ref : Inport
  Iq_ref : Inport  Port=2
  Complex to Magnitude-Angle : ComplexToMagnitudeAngle
  Complex to Real-Imag : ComplexToRealImag
  Magnitude-Angle to Complex : MagnitudeAngleToComplex
  Real-Imag to Complex : RealImagToComplex
  Saturation : Saturate  UpperLimit=Imax_solar2  LowerLimit=-Imax_solar2
  w3 : Scope  NumInputPorts=2
  Id_lim : Outport
  Iq_lim : Outport  Port=2
  wires:
  Complex to Magnitude-Angle/2 -> Magnitude-Angle to Complex/2
  Magnitude-Angle to Complex/1 -> Complex to Real-Imag/1
  Iq_ref/1 -> Real-Imag to Complex/2
  Id_ref/1 -> Real-Imag to Complex/1
  Complex to Magnitude-Angle/1 -> w3/1, Saturation/1
  Real-Imag to Complex/1 -> Complex to Magnitude-Angle/1
  Complex to Real-Imag/1 -> Id_lim/1
  Complex to Real-Imag/2 -> Iq_lim/1
  Saturation/1 -> w3/2, Magnitude-Angle to Complex/1

== matlab function MR_CIGRE_RESISTIVO/Banco de Baterias_2/Referência de Potencia/Referência Fonte ==
  settings: updateMethod=DISCRETE
  data: Pref_bat input; Qref_bat input; p input; Prefbat output; q input; Qrefbat output; Qr data_store_memory; Pr data_store_memory; sinc input
function [Prefbat,Qrefbat] = fcn(Pref_bat, Qref_bat, p, q,sinc)
global Qr;
global Pr;

    
if sinc==0
   Qrefbat=Qref_bat;      
   Prefbat=Pref_bat; 
   Qr = q;
   Pr = p;
else
    Qrefbat=Qr;
    Prefbat=Pr;
end
end

== matlab function MR_CIGRE_RESISTIVO/Sincronização/Função ==
  settings: updateMethod=DISCRETE
  data: t input; sinc output; T data_store_memory; sinc input; tsinc input
function sinc  = fcn(t,sinc,tsinc)
global T
T=t;

if (T>tsinc)||(sinc==1)
   if sinc==0   
      sinc=1;
   end 
end
end

== matlab function MR_CIGRE_RESISTIVO/Banco de Baterias_1/Referência de Potencia/Referência Fonte ==
  settings: updateMethod=DISCRETE
  data: Pref_bat input; Qref_bat input; p input; Prefbat output; q input; Qrefbat output; Qr data_store_memory; Pr data_store_memory; sinc input
function [Prefbat,Qrefbat] = fcn(Pref_bat, Qref_bat, p, q,sinc)
global Qr;
global Pr;

    
if sinc==0
   Qrefbat=Qref_bat;      
   Prefbat=Pref_bat; 
   Qr = q;
   Pr = p;
else
    Qrefbat=Qr;
    Prefbat=Pr;
end
end

== matlab function MR_CIGRE_RESISTIVO/Stop/StopSimulation ==
  settings: updateMethod=DISCRETE
  data: V input; Stop output; f input; P input; Q input; Int input; IntD input; Modo input; C data_store_memory
function Stop = fcn(V, f, P, Q, Int, IntD, Modo)
% Função para parar o simulink permitindo simulações em série
    global C
    MP = max(P);
    MQ = max(Q);
    if Modo == 1
        Stop = 0;
        C = 0;
    else
        if MP > 2 || MQ > 2 || V<0.4 || f < 0.4 || (C < Int-IntD && C > 5E-3)
            Stop = 1;
        else
            C = Int-IntD;
            Stop = 0;
        end
    end
end
